simulink model "SatSIM_revAgustus16_01_R2010a"  (Simulink 7.5)
settings: Solver=ode15s  StartTime=0.0  StopTime=6000  RelTol=1e-3
values from neighbouring files (symbols this model uses):
  dfy = d    [dfy.m]
  s = sin(ir)    [B_dipole_June16_2.m]    (also in LTC_to_NED.m = sin(e); LTC_to_NED_edit.m = sin(e); TimeConverter.m = fix(sec); read_epoch.m = ((e-h)*60)-min)
undefined symbols (not defined in the file or in its folder): B_dipole_June16_2, DCM_ROI, deg, Earth_MagField_may16_Rev4, InertiaMoment3, LTC_to_NED_edit, rad, read_epochS, sec_to_ymdhms2, SimpleB5
libraries: aerolibconvert2 x13, aerolibutil x7, simulink x5, aerolibtransform2 x4, dspmtrx3 x3, vrlib x2, aerolibanim x1
(part 2 of 2)

== matlab function Environtments/Transformation Coordinate/ECI to ECEF/teta between ECT and ECEF/Julian Date Formula at t ==
  data: days input double; month input double; years input double; hours input double; minutes input double; second input double; JD output double
function JD = JulianDate(days,month,years,hours,minutes,second)
%#eml
%dt = GMSt
%y=year
%m=month
%dy:days, date in the month
%h:hour
%mi:minute
%s:secon

%Initial value for calculating Julian Date
a=(14-month)/12;
y=years+4800-a; %number of year scinece March 1 -4800
m=month+(12*a)-3; %number of month scinece March 1 -4800

%Calculate Julian Date Number
JDN=days+(((153*m)+2)/5)+(365*y)+(y/4)-(y/100)+(y/400)-32045;

%Calculate Julian Date
J=JDN+((hours-12)/24)+(minutes/1440)+(second/86400);

JD = J;

== matlab function Environtments/Transformation Coordinate/ECI to ECEF/teta between ECT and ECEF/GMSt Formula 0 ==
  data: JD0 input double; GMSt0 output double
function GMSt0 = GMSt0(JD0)
%#eml
%GreenWich MeanSidereal Time or LST at GreenWich
%if give a UT (universal time)
%First, Calculate Julian Century or T
T0=(JD0-2451545)/36525;

%so, the GMSt given by
G0=24110.54841+(T0*8640184.812866)+((T0^2)*0.093104)-((T0^3)*0.0000062);
%in hours

GMSt0 = G0;

== matlab function Environtments/Transformation Coordinate/ECI to ECEF/teta between ECT and ECEF/Julian Date Formula at t0 ==
  data: days0 input double; month0 input double; years0 input double; hours0 input double; minutes0 input double; second0 input double; JD0 output double
function JD0 = JulianDate0(days0,month0,years0,hours0,minutes0,second0)
%#eml
%dt = GMSt
%y=year
%m=month
%dy:days, date in the month
%h:hour
%mi:minute
%s:secon

%Initial value for calculating Julian Date
a0=(14-month0)/12;
y0=years0+4800-a0; %number of year scinece March 1 -4800
m0=month0+(12*a0)-3; %number of month scinece March 1 -4800

%Calculate Julian Date Number
JDN0=days0+(((153*m0)+2)/5)+(365*y0)+(y0/4)-(y0/100)+(y0/400)-32045;

%Calculate Julian Date
J0=JDN0+((hours0-12)/24)+(minutes0/1440)+(second0/86400);

JD0 = J0;

== matlab function Environtments/Transformation Coordinate/ECEF to alt,lat,long/  ==
  data: lat input double; latitude output double
function latitude= fcn(lat)
%#eml
%jika sudut lebih besar dari 90 derajat maka
a=(abs(lat))/360;
if a<1
    latitude=abs(lat);
else
    b=fix(a);
    latitude=abs(lat-(b*360));
end
end

== matlab function Environtments/Transformation Coordinate/ECEF to alt,lat,long/    ==
  data: long input double; longitude output double
function longitude= fcn(long)
%#eml
%jika sudut lebih besar dari 360 derajat maka
%untuk sudut <360, sudut=sudut
%untuk sudut >360
a=(abs(long))/360;
if a<1
    longitude=abs(long);
else
    b=fix(a);
    longitude=abs(long-(b*360));
end
end

== matlab function Environtments/Transformation Coordinate/ECEF to NED/Matrix Rotation ECEF to Local Horizon ==
  data: Rlg output double; long input double; lat input double
function Rlg = RLG(long,lat)
%#eml
%alt = Altitude
%long = Longitude
%Lat = Latitude

%Matrix rotation from ECEF to Local Horizon
R1=[-sind(lat)*cosd(long) -sind(lat)*sind(long) cosd(lat);...
    -sind(long) cosd(long) 0;...
    -cosd(lat)*cosd(long) -cosd(lat)*sind(long) -sind(lat)];

Rlg = R1;

== matlab function Environtments/Transformation Coordinate/ECEF to alt,lat,long/alt,long,lat ==
  data: xG input double; alt output double; yG input double; zG input double; long output double; lat output double
function [alt, long, lat] = XYZtoALL(xG,yG,zG)
%#eml
%alttitude
alt=((xG^2)+(yG^2)+(zG^2))^0.5;

%longitude
long=atand(yG/xG);

%latitude
lat=atand(zG/(((xG^2)+(yG^2))^0.5));

end

== matlab function OUTPUT/date/s2hms ==
  data: secs input double; hour output double; min output double; sec output double
function [hour,min,sec]=s2hms(secs)
%S2HMS converts seconds to integer hour,minute,seconds
%
sec=round(secs);

h=fix(sec/3600);
if h<24
    hour=floor(sec/3600);
else
    a=fix((sec/3600)/24);
    hour=floor((sec/3600)-(24*a));
end

min=floor(rem(sec,3600)/60);
sec=round(rem(sec,60));
end

== matlab function Actuator/currents Y ==
  data: Imax input double; Ib output double; Iy input double
function Ib = currents(Imax,Iy)
%#Currents filter
if Iy>(-1*Imax) && Iy<Imax
    Ib=Iy;
else
    if Iy>0 %positif
        Ib=Imax;
    else % negatif
        Ib=-1*Imax;
    end
end
end

== matlab function Actuator/currents Z ==
  data: Imax input double; Ic output double; Iz input double
function Ic = currents(Imax,Iz)
%#Currents filter
if Iz>(-1*Imax) && Iz<Imax
    Ic=Iz;
else
    if Iz>0 %positif
        Ic=Imax;
    else % negatif
        Ic=-1*Imax;
    end
end
end

== matlab function dynamic inertial/w(t) to Quaternion/quaternion derivative ==
  data: q0 input double; q1 input double; q2 input double; q3 input double; qdot output double
function qdot   = q( q0,q1,q2,q3 )
%CONVERTION FROM ANGULAR VELOCITY TO QUATERNION
%-------------------------------------------------------------------------%
%   this block need and looping input and output so maybe there have a
%   singularities
%   OMG=angular velociti
%   with componen = [w1 w2 w3];
%   unit in degree/s
%   q have dimention 1x4, q=[q0 q1 q2 q3], q4=q0
%-------------------------------------------------------------------------%
%lets divine a matrix with dimention 4x3
qdot=[q0 -q3 q2;...
    q3 q0 -q1;...
    -q2 q1 q0;...
    -q1 -q2 -q3];
%--------------------------------END---------------------------------------%
end
